simulink model "watertank"  (Simulink 7.5)
settings: Solver=ode45  StartTime=0.0  StopTime=25  RelTol=1e-3
PreLoadFcn:
  | watertankdat
values from neighbouring files (symbols this model uses):
  a = 0.24    [Granulometria1.m]    (also in Granulometria10.m; Granulometria1a.m; Granulometria1fptHPGR5.m; Granulometria1m.m)
undefined symbols (not defined in the file or in its folder): A, b
libraries: simulink x1
settings Model: Creator=The MathWorks Inc.  LastModifiedBy=Fer
settings DataIOCC: SignalLoggingName=logsOut
settings OptimizationCC: InlineInvariantSignals=on  InitFltsAndDblsToZero=on
settings DebuggingCC: SaveWithParameterizedLinksMsg=none  SignalResolutionControl=TryResolveAllWithWarning  SolverPrmCheckMsg=none  MultiTaskDSMMsg=warning  StrictBusMsg=None
settings HardwareCC: ProdHWDeviceType=Specified
settings GRTTargetCC: TargetFcnLib=ansi_tfl_tmw.mat

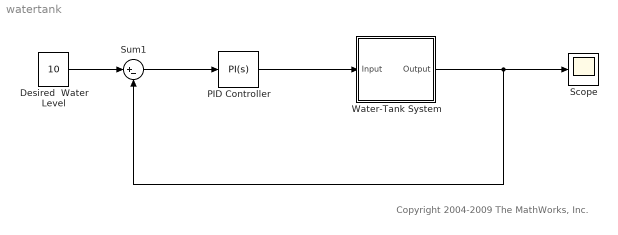
== system watertank ==
  note: Copyright 2004-2009 The MathWorks, Inc.
  Desired  Water Level : Constant  Value=10  OutDataType=sfix(16)  OutScaling=2^0
  PID Controller : simulink/Continuous/PID Controller  Tag=PID1  DialogController=pidpack.PIDConfig.pidDDGCreate  DialogControllerArgs=DataTag0  SystemSampleTime=-1  Controller=PI  TimeDomain=Continuous-time  SampleTime=1  IntegratorMethod=Forward Euler  FilterMethod=Forward Euler  Form=Parallel  P=1.599340  I=0.079967  D=-7.525674  N=0.201208  InitialConditionSource=internal  InitialConditionForIntegrator=0  InitialConditionForFilter=0  ExternalReset=none  ZeroCross=off  LimitOutput=off  UpperSaturationLimit=inf  LowerSaturationLimit=-inf  LinearizeAsGain=off  AntiWindupMode=none  Kb=1  TrackingMode=off  Kt=1  PParamMin=[ ]  PParamMax=[ ]  IParamMin=[ ]  IParamMax=[ ]  DParamMin=[ ]  DParamMax=[ ]  NParamMin=[ ]  NParamMax=[ ]  KbParamMin=[ ]  KbParamMax=[ ]  KtParamMin=[ ]  KtParamMax=[ ]  POutMin=[ ]  POutMax=[ ]  IOutMin=[ ]  IOutMax=[ ]  DOutMin=[ ]  DOutMax=[ ]  NOutMin=[ ]  NOutMax=[ ]  KbOutMin=[ ]  KbOutMax=[ ]  KtOutMin=[ ]  KtOutMax=[ ]  IntegratorOutMin=[ ]  IntegratorOutMax=[ ]  FilterOutMin=[ ]  FilterOutMax=[ ]  SumOutMin=[ ]  SumOutMax=[ ]  SumI1OutMin=[ ]  SumI1OutMax=[ ]  SumI2OutMin=[ ]  SumI2OutMax=[ ]  SumI3OutMin=[ ]  SumI3OutMax=[ ]  SumDOutMin=[ ]  SumDOutMax=[ ]  SaturationOutMin=[ ]  SaturationOutMax=[ ]  IntegratorContinuousStateAttributes=''  IntegratorStateMustResolveToSignalObject=off  IntegratorRTWStateStorageClass=Auto  FilterContinuousStateAttributes=''  FilterStateMustResolveToSignalObject=off  FilterRTWStateStorageClass=Auto
  Scope : Scope
  Sum1 : Sum  Inputs=|+-  OutDataType=sfix(16)  OutScaling=2^0  SaturateOnIntegerOverflow=on
  Water-Tank System : Subsystem
  wires:
  Desired  Water Level/1 -> Sum1/1
  Sum1/1 -> PID Controller/1
  Water-Tank System/1(Output) -> Sum1/2, Scope/1
  PID Controller/1 -> Water-Tank System/1(Input)

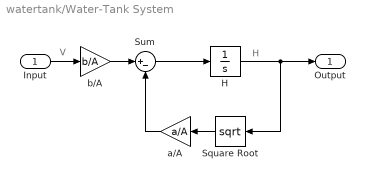
== system watertank/Water-Tank System ==
  note: H
  note: V
  Input : Inport  OutDataType=sfix(16)  OutScaling=2^0
  H : Integrator  InitialCondition=1
  Square Root : Math  Operator=sqrt  OutputSignalType=real  OutDataType=sfix(16)  OutScaling=2^0  SaturateOnIntegerOverflow=on
  Sum : Sum  Inputs=|+-  OutDataType=sfix(16)  OutScaling=2^0  SaturateOnIntegerOverflow=on
  a/A : Gain  Gain=a/A  ParameterDataType=sfix(16)  ParameterScaling=2^0  OutDataType=sfix(16)  OutScaling=2^0  SaturateOnIntegerOverflow=on  OutDataTypeStr=Inherit: Same as input  ParamDataTypeStr=Inherit: Same as input
  b/A : Gain  Gain=b/A  ParameterDataType=sfix(16)  ParameterScaling=2^0  OutDataType=sfix(16)  OutScaling=2^0  SaturateOnIntegerOverflow=on  OutDataTypeStr=Inherit: Same as input  ParamDataTypeStr=Inherit: Same as input
  Output : Outport  OutDataType=sfix(16)  OutScaling=2^0
  wires:
  b/A/1 -> Sum/1
  Sum/1 -> H/1
  H/1 -> Square Root/1, Output/1
  Square Root/1 -> a/A/1
  a/A/1 -> Sum/2
  Input/1 -> b/A/1
